simulink model "MIL4L3_SW6_V1_20220211"  (R2018b)
settings: Solver=FixedStepAuto  StartTime=0.0  StopTime=inf  FixedStep=0.001  RelTol=1e-3
PreLoadFcn:
  | A0_MILtest;
undefined symbols (not defined in the file or in its folder): Clb_ICADirect_LaneDisp_StateFive, Clb_ICADirect_LaneDisp_StateFour, Clb_ICADirect_LaneDisp_StateOne, Clb_ICADirect_LaneDisp_StateThree, Clb_ICADirect_LaneDisp_StateTwo, Clb_ICADirect_LaneDisp_StateZero, Clb_ICADirect_LaneDispSW, Clb_ICADirect_TrnLghtsCom_Switch, Clb_ICADirect_TrnLghtsCom_Value, Clb_ICADirect_TrnLghtsCrtl_Inhb, IMAP_Clb_ACU_Driver_Belt, IMAP_Clb_ACU_Driver_Belt_Over, IMAP_Clb_ACU_Passenger_Belt, IMAP_Clb_ACU_Passenger_Belt_Over, IMAP_Clb_ACU_RearLeft_Belt, IMAP_Clb_ACU_RearLeft_Belt_Over, IMAP_Clb_ACU_RearMiddle_Belt, IMAP_Clb_ACU_RearMiddle_Belt_Over, IMAP_Clb_ACU_RearRight_Belt, IMAP_Clb_ACU_RearRight_Belt_Over, IMAP_Clb_AEB_Switch, IMAP_Clb_AEB_Switch_Over, IMAP_Clb_ALC_TLC_Mode, IMAP_Clb_ALC_TLC_Mode_Over, IMAP_Clb_BCM_Battery_Voltage, IMAP_Clb_BCM_Battery_Voltage_Over, IMAP_Clb_BCM_BrakeLamp_State, IMAP_Clb_BCM_BrakeLamp_State_Over, IMAP_Clb_BCM_CHMSL_Status, IMAP_Clb_BCM_CHMSL_Status_Over, IMAP_Clb_BCM_Door_Lock_State, IMAP_Clb_BCM_Door_Lock_State_Over, IMAP_Clb_BCM_FrontWiper_State, IMAP_Clb_BCM_FrontWiper_State_Over, IMAP_Clb_BCM_FrontWiper_Switch, IMAP_Clb_BCM_FrontWiper_Switch_Over, IMAP_Clb_BCM_HazardLamp, IMAP_Clb_BCM_HazardLamp_Over, IMAP_Clb_BCM_HazardLamp_Switch, IMAP_Clb_BCM_HazardLamp_Switch_Over, IMAP_Clb_BCM_HighBeam_State, IMAP_Clb_BCM_HighBeam_State_Over, IMAP_Clb_BCM_Ignition_State, IMAP_Clb_BCM_Ignition_State_Over, IMAP_Clb_BCM_IHBC_Enabled, IMAP_Clb_BCM_IHBC_Enabled_Over, IMAP_Clb_BCM_Left_Light, IMAP_Clb_BCM_Left_Light_Over, IMAP_Clb_BCM_LeftTurn_Switch, IMAP_Clb_BCM_LeftTurn_Switch_Over, IMAP_Clb_BCM_LF_Door_State, IMAP_Clb_BCM_LF_Door_State_Over, IMAP_Clb_BCM_LowBeam_State, IMAP_Clb_BCM_LowBeam_State_Over, IMAP_Clb_BCM_LR_Door_State, IMAP_Clb_BCM_LR_Door_State_Over, IMAP_Clb_BCM_RF_Door_State, IMAP_Clb_BCM_RF_Door_State_Over, IMAP_Clb_BCM_Right_Light, IMAP_Clb_BCM_Right_Light_Over ... (+547)
libraries: CarMaker4SL x2153, simulink x292, dspstat3 x3, canmsglib x2, simulink_extras x1
(part 15 of 52)

== system MIL4L3_SW6_V1_20220211/CarMaker/VehicleControl/SDFADataLog/Subsystem113 ==
  BusCreator : BusCreator  Inputs=10
  Data Type Conversion{1..3,92} (4 alike) : DataTypeConversion  OutDataTypeStr=single
  Ground{,1..5} (6 alike) : Ground
  Read CM Dict1 : CarMaker4SL/Read CM Dict  xname=User.IO.Out.YAcceleration_S1_002  xsync=off
  Read CM Dict2 : CarMaker4SL/Read CM Dict  xname=User.IO.Out.YAcceleration_S1_003  xsync=off
  Read CM Dict3 : CarMaker4SL/Read CM Dict  xname=User.IO.Out.YAcceleration_S1_004  xsync=off
  Read CM Dict5 : CarMaker4SL/Read CM Dict  xname=User.IO.Out.YAcceleration_S1_001  xsync=off
  RBtar_Yacceleration : Outport
  wires:
  Data Type Conversion1/1 -> BusCreator/2
  Data Type Conversion92/1 -> BusCreator/1
  Data Type Conversion3/1 -> BusCreator/4
  Data Type Conversion2/1 -> BusCreator/3
  BusCreator/1 -> RBtar_Yacceleration/1
  Read CM Dict3/1 -> Data Type Conversion3/1
  Read CM Dict2/1 -> Data Type Conversion2/1
  Read CM Dict1/1 -> Data Type Conversion1/1
  Read CM Dict5/1 -> Data Type Conversion92/1
  Ground/1 -> BusCreator/5
  Ground1/1 -> BusCreator/6
  Ground2/1 -> BusCreator/7
  Ground3/1 -> BusCreator/8
  Ground4/1 -> BusCreator/9
  Ground5/1 -> BusCreator/10

== system MIL4L3_SW6_V1_20220211/CarMaker/VehicleControl/SDFADataLog/Subsystem114 ==
  BusCreator : BusCreator  Inputs=10
  Data Type Conversion{1..3,92} (4 alike) : DataTypeConversion  OutDataTypeStr=single
  Ground{,1..5} (6 alike) : Ground
  Read CM Dict1 : CarMaker4SL/Read CM Dict  xname=User.IO.Out.Width_S1_002  xsync=off
  Read CM Dict2 : CarMaker4SL/Read CM Dict  xname=User.IO.Out.Width_S1_003  xsync=off
  Read CM Dict3 : CarMaker4SL/Read CM Dict  xname=User.IO.Out.Width_S1_004  xsync=off
  Read CM Dict5 : CarMaker4SL/Read CM Dict  xname=User.IO.Out.Width_S1_001  xsync=off
  RBtar_Width : Outport
  wires:
  Data Type Conversion2/1 -> BusCreator/3
  Data Type Conversion3/1 -> BusCreator/4
  Data Type Conversion1/1 -> BusCreator/2
  Data Type Conversion92/1 -> BusCreator/1
  Ground5/1 -> BusCreator/10
  Ground4/1 -> BusCreator/9
  Ground3/1 -> BusCreator/8
  Ground2/1 -> BusCreator/7
  Ground1/1 -> BusCreator/6
  Ground/1 -> BusCreator/5
  Read CM Dict5/1 -> Data Type Conversion92/1
  Read CM Dict1/1 -> Data Type Conversion1/1
  Read CM Dict2/1 -> Data Type Conversion2/1
  Read CM Dict3/1 -> Data Type Conversion3/1
  BusCreator/1 -> RBtar_Width/1

== system MIL4L3_SW6_V1_20220211/CarMaker/VehicleControl/SDFADataLog/Subsystem115 ==
  BusCreator : BusCreator  Inputs=10
  Data Type Conversion{1..3,92} (4 alike) : DataTypeConversion  OutDataTypeStr=single
  Ground{,1..5} (6 alike) : Ground
  Read CM Dict1 : CarMaker4SL/Read CM Dict  xname=User.IO.Out.Length_S1_002  xsync=off
  Read CM Dict2 : CarMaker4SL/Read CM Dict  xname=User.IO.Out.Length_S1_003  xsync=off
  Read CM Dict3 : CarMaker4SL/Read CM Dict  xname=User.IO.Out.Length_S1_004  xsync=off
  Read CM Dict5 : CarMaker4SL/Read CM Dict  xname=User.IO.Out.Length_S1_001  xsync=off
  RBtar_Length : Outport
  wires:
  Data Type Conversion2/1 -> BusCreator/3
  Data Type Conversion3/1 -> BusCreator/4
  Data Type Conversion92/1 -> BusCreator/1
  Data Type Conversion1/1 -> BusCreator/2
  BusCreator/1 -> RBtar_Length/1
  Read CM Dict3/1 -> Data Type Conversion3/1
  Read CM Dict2/1 -> Data Type Conversion2/1
  Read CM Dict1/1 -> Data Type Conversion1/1
  Read CM Dict5/1 -> Data Type Conversion92/1
  Ground/1 -> BusCreator/5
  Ground1/1 -> BusCreator/6
  Ground2/1 -> BusCreator/7
  Ground3/1 -> BusCreator/8
  Ground4/1 -> BusCreator/9
  Ground5/1 -> BusCreator/10

== system MIL4L3_SW6_V1_20220211/CarMaker/VehicleControl/SDFADataLog/Subsystem116 ==
  BusCreator : BusCreator  Inputs=10
  Data Type Conversion{1..3,92} (4 alike) : DataTypeConversion  OutDataTypeStr=single
  Ground{,1..5} (6 alike) : Ground
  Read CM Dict1 : CarMaker4SL/Read CM Dict  xname=User.IO.Out.Orientation_S1_002  xsync=off
  Read CM Dict2 : CarMaker4SL/Read CM Dict  xname=User.IO.Out.Orientation_S1_003  xsync=off
  Read CM Dict3 : CarMaker4SL/Read CM Dict  xname=User.IO.Out.Orientation_S1_004  xsync=off
  Read CM Dict5 : CarMaker4SL/Read CM Dict  xname=User.IO.Out.Orientation_S1_001  xsync=off
  RBtar_Orientation : Outport
  wires:
  Data Type Conversion92/1 -> BusCreator/1
  Data Type Conversion3/1 -> BusCreator/4
  Data Type Conversion2/1 -> BusCreator/3
  Data Type Conversion1/1 -> BusCreator/2
  Ground5/1 -> BusCreator/10
  Ground4/1 -> BusCreator/9
  Ground3/1 -> BusCreator/8
  Ground2/1 -> BusCreator/7
  Ground1/1 -> BusCreator/6
  Ground/1 -> BusCreator/5
  Read CM Dict5/1 -> Data Type Conversion92/1
  Read CM Dict1/1 -> Data Type Conversion1/1
  Read CM Dict2/1 -> Data Type Conversion2/1
  Read CM Dict3/1 -> Data Type Conversion3/1
  BusCreator/1 -> RBtar_Orientation/1

== system MIL4L3_SW6_V1_20220211/CarMaker/VehicleControl/SDFADataLog/Subsystem117 ==
  BusCreator : BusCreator  Inputs=10
  Data Type Conversion{1..3,92} (4 alike) : DataTypeConversion  OutDataTypeStr=single
  Ground{,1..5} (6 alike) : Ground
  Read CM Dict1 : CarMaker4SL/Read CM Dict  xname=User.IO.Out.ExistenceProbability_S1_002  xsync=off
  Read CM Dict2 : CarMaker4SL/Read CM Dict  xname=User.IO.Out.ExistenceProbability_S1_003  xsync=off
  Read CM Dict3 : CarMaker4SL/Read CM Dict  xname=User.IO.Out.ExistenceProbability_S1_004  xsync=off
  Read CM Dict5 : CarMaker4SL/Read CM Dict  xname=User.IO.Out.ExistenceProbability_S1_001  xsync=off
  RBtar_ExistenceProbability : Outport
  wires:
  Data Type Conversion3/1 -> BusCreator/4
  Data Type Conversion2/1 -> BusCreator/3
  Data Type Conversion92/1 -> BusCreator/1
  Data Type Conversion1/1 -> BusCreator/2
  BusCreator/1 -> RBtar_ExistenceProbability/1
  Read CM Dict3/1 -> Data Type Conversion3/1
  Read CM Dict2/1 -> Data Type Conversion2/1
  Read CM Dict1/1 -> Data Type Conversion1/1
  Read CM Dict5/1 -> Data Type Conversion92/1
  Ground/1 -> BusCreator/5
  Ground1/1 -> BusCreator/6
  Ground2/1 -> BusCreator/7
  Ground3/1 -> BusCreator/8
  Ground4/1 -> BusCreator/9
  Ground5/1 -> BusCreator/10

== system MIL4L3_SW6_V1_20220211/CarMaker/VehicleControl/SDFADataLog/Subsystem118 ==
  BusCreator : BusCreator  Inputs=10
  Data Type Conversion{1..3,92} (4 alike) : DataTypeConversion  OutDataTypeStr=uint8
  Ground{,1..5} (6 alike) : Ground
  Read CM Dict1 : CarMaker4SL/Read CM Dict  xname=User.IO.Out.ClassHighest_S1_002  xsync=off
  Read CM Dict2 : CarMaker4SL/Read CM Dict  xname=User.IO.Out.ClassHighest_S1_003  xsync=off
  Read CM Dict3 : CarMaker4SL/Read CM Dict  xname=User.IO.Out.ClassHighest_S1_004  xsync=off
  Read CM Dict5 : CarMaker4SL/Read CM Dict  xname=User.IO.Out.ClassHighest_S1_001  xsync=off
  RBtar_Class : Outport
  wires:
  Data Type Conversion1/1 -> BusCreator/2
  Data Type Conversion2/1 -> BusCreator/3
  Data Type Conversion3/1 -> BusCreator/4
  Data Type Conversion92/1 -> BusCreator/1
  Ground5/1 -> BusCreator/10
  Ground4/1 -> BusCreator/9
  Ground3/1 -> BusCreator/8
  Ground2/1 -> BusCreator/7
  Ground1/1 -> BusCreator/6
  Ground/1 -> BusCreator/5
  Read CM Dict5/1 -> Data Type Conversion92/1
  Read CM Dict1/1 -> Data Type Conversion1/1
  Read CM Dict2/1 -> Data Type Conversion2/1
  Read CM Dict3/1 -> Data Type Conversion3/1
  BusCreator/1 -> RBtar_Class/1

== system MIL4L3_SW6_V1_20220211/CarMaker/VehicleControl/SDFADataLog/Subsystem119 ==
  BusCreator : BusCreator  Inputs=10
  Data Type Conversion{1..3,92} (4 alike) : DataTypeConversion  OutDataTypeStr=single
  Ground{,1..5} (6 alike) : Ground
  Read CM Dict1 : CarMaker4SL/Read CM Dict  xname=User.IO.Out.ReferencePoint_S1_002  xsync=off
  Read CM Dict2 : CarMaker4SL/Read CM Dict  xname=User.IO.Out.ReferencePoint_S1_003  xsync=off
  Read CM Dict3 : CarMaker4SL/Read CM Dict  xname=User.IO.Out.ReferencePoint_S1_004  xsync=off
  Read CM Dict5 : CarMaker4SL/Read CM Dict  xname=User.IO.Out.ReferencePoint_S1_001  xsync=off
  RBtar_ReferencePoint : Outport
  wires:
  Data Type Conversion3/1 -> BusCreator/4
  Data Type Conversion2/1 -> BusCreator/3
  Data Type Conversion92/1 -> BusCreator/1
  Data Type Conversion1/1 -> BusCreator/2
  BusCreator/1 -> RBtar_ReferencePoint/1
  Read CM Dict3/1 -> Data Type Conversion3/1
  Read CM Dict2/1 -> Data Type Conversion2/1
  Read CM Dict1/1 -> Data Type Conversion1/1
  Read CM Dict5/1 -> Data Type Conversion92/1
  Ground/1 -> BusCreator/5
  Ground1/1 -> BusCreator/6
  Ground2/1 -> BusCreator/7
  Ground3/1 -> BusCreator/8
  Ground4/1 -> BusCreator/9
  Ground5/1 -> BusCreator/10

== system MIL4L3_SW6_V1_20220211/CarMaker/VehicleControl/SDFADataLog/Subsystem12 ==
  Bus Creator : BusCreator  Inputs=20
  Ground{,1..15} (16 alike) : Ground
  Read CM Dict : CarMaker4SL/Read CM Dict  xname=User.IO.Out.IFC_obj01_Rel_VxStdDevValid  xsync=off
  Read CM Dict1 : CarMaker4SL/Read CM Dict  xname=User.IO.Out.IFC_obj02_Rel_VxStdDevValid  xsync=off
  Read CM Dict2 : CarMaker4SL/Read CM Dict  xname=User.IO.Out.IFC_obj03_Rel_VxStdDevValid  xsync=off
  Read CM Dict3 : CarMaker4SL/Read CM Dict  xname=User.IO.Out.IFC_obj04_Rel_VxStdDevValid  xsync=off
  obj_Rel_VxStdDevValid : Outport
  wires:
  Bus Creator/1 -> obj_Rel_VxStdDevValid/1
  Ground15/1 -> Bus Creator/20
  Ground11/1 -> Bus Creator/16
  Ground14/1 -> Bus Creator/19
  Ground12/1 -> Bus Creator/17
  Ground3/1 -> Bus Creator/8
  Ground1/1 -> Bus Creator/6
  Read CM Dict1/1 -> Bus Creator/2
  Read CM Dict/1 -> Bus Creator/1
  Ground6/1 -> Bus Creator/11
  Ground10/1 -> Bus Creator/15
  Ground13/1 -> Bus Creator/18
  Ground2/1 -> Bus Creator/7
  Ground/1 -> Bus Creator/5
  Ground7/1 -> Bus Creator/12
  Read CM Dict3/1 -> Bus Creator/4
  Ground4/1 -> Bus Creator/9
  Ground9/1 -> Bus Creator/14
  Ground5/1 -> Bus Creator/10
  Ground8/1 -> Bus Creator/13
  Read CM Dict2/1 -> Bus Creator/3

== system MIL4L3_SW6_V1_20220211/CarMaker/VehicleControl/SDFADataLog/Subsystem120 ==
  BusCreator : BusCreator  Inputs=10
  Data Type Conversion{1..3,92} (4 alike) : DataTypeConversion  OutDataTypeStr=single
  Ground{,1..5} (6 alike) : Ground
  Read CM Dict1 : CarMaker4SL/Read CM Dict  xname=User.IO.Out.MovingState_S1_002  xsync=off
  Read CM Dict2 : CarMaker4SL/Read CM Dict  xname=User.IO.Out.MovingState_S1_003  xsync=off
  Read CM Dict3 : CarMaker4SL/Read CM Dict  xname=User.IO.Out.MovingState_S1_004  xsync=off
  Read CM Dict5 : CarMaker4SL/Read CM Dict  xname=User.IO.Out.MovingState_S1_001  xsync=off
  RBtar_MovingState : Outport
  wires:
  Data Type Conversion2/1 -> BusCreator/3
  Data Type Conversion92/1 -> BusCreator/1
  Data Type Conversion3/1 -> BusCreator/4
  Data Type Conversion1/1 -> BusCreator/2
  Ground5/1 -> BusCreator/10
  Ground4/1 -> BusCreator/9
  Ground3/1 -> BusCreator/8
  Ground2/1 -> BusCreator/7
  Ground1/1 -> BusCreator/6
  Ground/1 -> BusCreator/5
  Read CM Dict5/1 -> Data Type Conversion92/1
  Read CM Dict1/1 -> Data Type Conversion1/1
  Read CM Dict2/1 -> Data Type Conversion2/1
  Read CM Dict3/1 -> Data Type Conversion3/1
  BusCreator/1 -> RBtar_MovingState/1

== system MIL4L3_SW6_V1_20220211/CarMaker/VehicleControl/SDFADataLog/Subsystem13 ==
  BusCreator : BusCreator  Inputs=24
  Constant{,1..3} (4 alike) : Constant  Value=0
  Ground{,1..19} (20 alike) : Ground
  Read CM Dict : CarMaker4SL/Read CM Dict  Commented=on  xname=User.IO.Out.BrakingAllowed_00  xsync=off
  Read CM Dict1 : CarMaker4SL/Read CM Dict  Commented=on  xname=User.IO.Out.BrakingAllowed_01  xsync=off
  Read CM Dict2 : CarMaker4SL/Read CM Dict  Commented=on  xname=User.IO.Out.BrakingAllowed_02  xsync=off
  Read CM Dict3 : CarMaker4SL/Read CM Dict  Commented=on  xname=User.IO.Out.BrakingAllowed_03  xsync=off
  BrakingAllowed : Outport
  wires:
  Constant3/1 -> BusCreator/4
  Ground19/1 -> BusCreator/24
  Ground18/1 -> BusCreator/23
  Ground5/1 -> BusCreator/10
  Ground3/1 -> BusCreator/8
  Ground9/1 -> BusCreator/14
  BusCreator/1 -> BrakingAllowed/1
  Ground11/1 -> BusCreator/16
  Ground8/1 -> BusCreator/13
  Ground7/1 -> BusCreator/12
  Ground15/1 -> BusCreator/18
  Ground1/1 -> BusCreator/6
  Ground/1 -> BusCreator/5
  Ground13/1 -> BusCreator/22
  Ground4/1 -> BusCreator/9
  Ground17/1 -> BusCreator/20
  Constant/1 -> BusCreator/1
  Ground10/1 -> BusCreator/15
  Constant2/1 -> BusCreator/3
  Ground6/1 -> BusCreator/11
  Constant1/1 -> BusCreator/2
  Ground2/1 -> BusCreator/7
  Ground14/1 -> BusCreator/17
  Ground16/1 -> BusCreator/19
  Ground12/1 -> BusCreator/21

== system MIL4L3_SW6_V1_20220211/CarMaker/VehicleControl/SDFADataLog/Subsystem14 ==
  BusCreator : BusCreator  Inputs=24
  Ground{,1..19} (20 alike) : Ground
  Read CM Dict : CarMaker4SL/Read CM Dict  xname=User.IO.Out.RadarCrossSection_00  xsync=off
  Read CM Dict1 : CarMaker4SL/Read CM Dict  xname=User.IO.Out.RadarCrossSection_01  xsync=off
  Read CM Dict2 : CarMaker4SL/Read CM Dict  xname=User.IO.Out.RadarCrossSection_02  xsync=off
  Read CM Dict3 : CarMaker4SL/Read CM Dict  xname=User.IO.Out.RadarCrossSection_03  xsync=off
  RadarCrossSection : Outport
  wires:
  Ground12/1 -> BusCreator/21
  Ground16/1 -> BusCreator/19
  Ground14/1 -> BusCreator/17
  Ground2/1 -> BusCreator/7
  Read CM Dict1/1 -> BusCreator/2
  Ground6/1 -> BusCreator/11
  Read CM Dict2/1 -> BusCreator/3
  Ground10/1 -> BusCreator/15
  Read CM Dict/1 -> BusCreator/1
  Ground17/1 -> BusCreator/20
  Ground4/1 -> BusCreator/9
  Ground13/1 -> BusCreator/22
  Ground/1 -> BusCreator/5
  Ground1/1 -> BusCreator/6
  Ground15/1 -> BusCreator/18
  Ground7/1 -> BusCreator/12
  Ground8/1 -> BusCreator/13
  Ground11/1 -> BusCreator/16
  BusCreator/1 -> RadarCrossSection/1
  Ground9/1 -> BusCreator/14
  Ground3/1 -> BusCreator/8
  Ground5/1 -> BusCreator/10
  Ground18/1 -> BusCreator/23
  Ground19/1 -> BusCreator/24
  Read CM Dict3/1 -> BusCreator/4

== system MIL4L3_SW6_V1_20220211/CarMaker/VehicleControl/SDFADataLog/Subsystem149 ==
  Bus Creator : BusCreator  Inputs=20
  Ground{,1..15} (16 alike) : Ground
  Read CM Dict : CarMaker4SL/Read CM Dict  xname=User.IO.Out.IFC_obj01_ExistProb  xsync=off
  Read CM Dict1 : CarMaker4SL/Read CM Dict  xname=User.IO.Out.IFC_obj02_ExistProb  xsync=off
  Read CM Dict2 : CarMaker4SL/Read CM Dict  xname=User.IO.Out.IFC_obj03_ExistProb  xsync=off
  Read CM Dict3 : CarMaker4SL/Read CM Dict  xname=User.IO.Out.IFC_obj04_ExistProb  xsync=off
  obj_ExistProb : Outport
  wires:
  Bus Creator/1 -> obj_ExistProb/1
  Ground15/1 -> Bus Creator/20
  Ground11/1 -> Bus Creator/16
  Ground14/1 -> Bus Creator/19
  Ground12/1 -> Bus Creator/17
  Ground3/1 -> Bus Creator/8
  Ground1/1 -> Bus Creator/6
  Read CM Dict1/1 -> Bus Creator/2
  Read CM Dict/1 -> Bus Creator/1
  Ground6/1 -> Bus Creator/11
  Ground10/1 -> Bus Creator/15
  Ground13/1 -> Bus Creator/18
  Ground2/1 -> Bus Creator/7
  Ground/1 -> Bus Creator/5
  Ground7/1 -> Bus Creator/12
  Read CM Dict3/1 -> Bus Creator/4
  Ground4/1 -> Bus Creator/9
  Ground9/1 -> Bus Creator/14
  Ground5/1 -> Bus Creator/10
  Ground8/1 -> Bus Creator/13
  Read CM Dict2/1 -> Bus Creator/3

== system MIL4L3_SW6_V1_20220211/CarMaker/VehicleControl/SDFADataLog/Subsystem150 ==
  BusCreator : BusCreator  Inputs=24
  Ground{,1..19} (20 alike) : Ground
  Read CM Dict : CarMaker4SL/Read CM Dict  xname=User.IO.Out.AbsoluteLongAcc_00  xsync=off
  Read CM Dict1 : CarMaker4SL/Read CM Dict  xname=User.IO.Out.AbsoluteLongAcc_01  xsync=off
  Read CM Dict2 : CarMaker4SL/Read CM Dict  xname=User.IO.Out.AbsoluteLongAcc_02  xsync=off
  Read CM Dict3 : CarMaker4SL/Read CM Dict  xname=User.IO.Out.AbsoluteLongAcc_03  xsync=off
  AbsoluteLongAcc : Outport
  wires:
  Ground12/1 -> BusCreator/21
  Ground16/1 -> BusCreator/19
  Ground14/1 -> BusCreator/17
  Ground2/1 -> BusCreator/7
  Read CM Dict1/1 -> BusCreator/2
  Ground6/1 -> BusCreator/11
  Read CM Dict2/1 -> BusCreator/3
  Ground10/1 -> BusCreator/15
  Read CM Dict/1 -> BusCreator/1
  Ground17/1 -> BusCreator/20
  Ground4/1 -> BusCreator/9
  Ground13/1 -> BusCreator/22
  Ground/1 -> BusCreator/5
  Ground1/1 -> BusCreator/6
  Ground15/1 -> BusCreator/18
  Ground7/1 -> BusCreator/12
  Ground8/1 -> BusCreator/13
  Ground11/1 -> BusCreator/16
  BusCreator/1 -> AbsoluteLongAcc/1
  Ground9/1 -> BusCreator/14
  Ground3/1 -> BusCreator/8
  Ground5/1 -> BusCreator/10
  Ground18/1 -> BusCreator/23
  Ground19/1 -> BusCreator/24
  Read CM Dict3/1 -> BusCreator/4

== system MIL4L3_SW6_V1_20220211/CarMaker/VehicleControl/SDFADataLog/Subsystem160 ==
  Bus Creator : BusCreator  Inputs=20
  Ground{,1..15} (16 alike) : Ground
  Read CM Dict : CarMaker4SL/Read CM Dict  xname=User.IO.Out.IFC_obj01_Rel_Vx  xsync=off
  Read CM Dict1 : CarMaker4SL/Read CM Dict  xname=User.IO.Out.IFC_obj02_Rel_Vx  xsync=off
  Read CM Dict2 : CarMaker4SL/Read CM Dict  xname=User.IO.Out.IFC_obj03_Rel_Vx  xsync=off
  Read CM Dict3 : CarMaker4SL/Read CM Dict  xname=User.IO.Out.IFC_obj04_Rel_Vx  xsync=off
  obj_Rel_Vx : Outport
  wires:
  Bus Creator/1 -> obj_Rel_Vx/1
  Ground15/1 -> Bus Creator/20
  Ground11/1 -> Bus Creator/16
  Ground14/1 -> Bus Creator/19
  Ground12/1 -> Bus Creator/17
  Ground3/1 -> Bus Creator/8
  Ground1/1 -> Bus Creator/6
  Read CM Dict1/1 -> Bus Creator/2
  Read CM Dict/1 -> Bus Creator/1
  Ground6/1 -> Bus Creator/11
  Ground10/1 -> Bus Creator/15
  Ground13/1 -> Bus Creator/18
  Ground2/1 -> Bus Creator/7
  Ground/1 -> Bus Creator/5
  Ground7/1 -> Bus Creator/12
  Read CM Dict3/1 -> Bus Creator/4
  Ground4/1 -> Bus Creator/9
  Ground9/1 -> Bus Creator/14
  Ground5/1 -> Bus Creator/10
  Ground8/1 -> Bus Creator/13
  Read CM Dict2/1 -> Bus Creator/3

== system MIL4L3_SW6_V1_20220211/CarMaker/VehicleControl/SDFADataLog/Subsystem171 ==
  Bus Creator : BusCreator  Inputs=20
  Ground{,1..15} (16 alike) : Ground
  Read CM Dict : CarMaker4SL/Read CM Dict  xname=User.IO.Out.IFC_obj01_Rel_VxValid  xsync=off
  Read CM Dict1 : CarMaker4SL/Read CM Dict  xname=User.IO.Out.IFC_obj02_Rel_VxValid  xsync=off
  Read CM Dict2 : CarMaker4SL/Read CM Dict  xname=User.IO.Out.IFC_obj03_Rel_VxValid  xsync=off
  Read CM Dict3 : CarMaker4SL/Read CM Dict  xname=User.IO.Out.IFC_obj04_Rel_VxValid  xsync=off
  obj_Rel_VxValid : Outport
  wires:
  Bus Creator/1 -> obj_Rel_VxValid/1
  Ground15/1 -> Bus Creator/20
  Ground11/1 -> Bus Creator/16
  Ground14/1 -> Bus Creator/19
  Ground12/1 -> Bus Creator/17
  Ground3/1 -> Bus Creator/8
  Ground1/1 -> Bus Creator/6
  Read CM Dict1/1 -> Bus Creator/2
  Read CM Dict/1 -> Bus Creator/1
  Ground6/1 -> Bus Creator/11
  Ground10/1 -> Bus Creator/15
  Ground13/1 -> Bus Creator/18
  Ground2/1 -> Bus Creator/7
  Ground/1 -> Bus Creator/5
  Ground7/1 -> Bus Creator/12
  Read CM Dict3/1 -> Bus Creator/4
  Ground4/1 -> Bus Creator/9
  Ground9/1 -> Bus Creator/14
  Ground5/1 -> Bus Creator/10
  Ground8/1 -> Bus Creator/13
  Read CM Dict2/1 -> Bus Creator/3

== system MIL4L3_SW6_V1_20220211/CarMaker/VehicleControl/SDFADataLog/Subsystem174 ==
  BusCreator : BusCreator  Inputs=24
  Constant{1..4} (4 alike) : Constant  Value=0.01
  Define CM Dict_User.IO.Out.LateralDistanceSTD_00 : CarMaker4SL/Define CM Dict  Commented=on  xname=User.IO.Out.LateralDistanceSTD_00  xunit=m  xmono=off  xtype=Double4  xdvaplace=IO_Out  xnstates=0  xfirststate=0  xinitial=0
  Ground{,1..19} (20 alike) : Ground
  LateralDistanceSTD : Outport
  wires:
  Ground18/1 -> BusCreator/23
  Ground19/1 -> BusCreator/24
  BusCreator/1 -> LateralDistanceSTD/1
  Ground8/1 -> BusCreator/13
  Ground5/1 -> BusCreator/10
  Ground3/1 -> BusCreator/8
  Ground/1 -> BusCreator/5
  Ground6/1 -> BusCreator/11
  Ground7/1 -> BusCreator/12
  Ground1/1 -> BusCreator/6
  Ground9/1 -> BusCreator/14
  Ground10/1 -> BusCreator/15
  Ground11/1 -> BusCreator/16
  Ground15/1 -> BusCreator/18
  Ground4/1 -> BusCreator/9
  Ground13/1 -> BusCreator/22
  Ground12/1 -> BusCreator/21
  Ground14/1 -> BusCreator/17
  Ground17/1 -> BusCreator/20
  Ground2/1 -> BusCreator/7
  Ground16/1 -> BusCreator/19
  Constant1/1 -> BusCreator/1
  Constant2/1 -> BusCreator/2
  Constant3/1 -> BusCreator/3
  Constant4/1 -> BusCreator/4

== system MIL4L3_SW6_V1_20220211/CarMaker/VehicleControl/SDFADataLog/Subsystem175 ==
  BusCreator : BusCreator  Inputs=24
  Constant{1..4} (4 alike) : Constant  Value=0.01
  Define CM Dict_User.IO.Out.LongDistanceSTD_00 : CarMaker4SL/Define CM Dict  Commented=on  xname=User.IO.Out.LongDistanceSTD_00  xunit=m  xmono=off  xtype=Double4  xdvaplace=IO_Out  xnstates=0  xfirststate=0  xinitial=0
  Ground{,1..19} (20 alike) : Ground
  Read CM Dict : CarMaker4SL/Read CM Dict  Commented=on  xname=User.IO.Out.LongDistance_00  xsync=off
  LongDistanceSTD : Outport
  wires:
  Constant4/1 -> BusCreator/4
  Constant3/1 -> BusCreator/3
  Constant2/1 -> BusCreator/2
  Constant1/1 -> BusCreator/1
  Ground16/1 -> BusCreator/19
  Ground2/1 -> BusCreator/7
  Ground17/1 -> BusCreator/20
  Ground14/1 -> BusCreator/17
  Ground12/1 -> BusCreator/21
  Ground13/1 -> BusCreator/22
  Ground4/1 -> BusCreator/9
  Ground15/1 -> BusCreator/18
  Ground11/1 -> BusCreator/16
  Ground10/1 -> BusCreator/15
  Ground9/1 -> BusCreator/14
  Ground1/1 -> BusCreator/6
  Ground7/1 -> BusCreator/12
  Ground6/1 -> BusCreator/11
  Ground/1 -> BusCreator/5
  Ground3/1 -> BusCreator/8
  Ground5/1 -> BusCreator/10
  Ground8/1 -> BusCreator/13
  BusCreator/1 -> LongDistanceSTD/1
  Ground19/1 -> BusCreator/24
  Ground18/1 -> BusCreator/23

== system MIL4L3_SW6_V1_20220211/CarMaker/VehicleControl/SDFADataLog/Subsystem176 ==
  BusCreator : BusCreator  Inputs=24
  Constant{,1..3} (4 alike) : Constant  Value=0.01
  Ground{,1..19} (20 alike) : Ground
  AbsoluteLongAccSTD : Outport
  wires:
  Constant3/1 -> BusCreator/4
  Ground19/1 -> BusCreator/24
  Ground18/1 -> BusCreator/23
  Ground5/1 -> BusCreator/10
  Ground3/1 -> BusCreator/8
  Ground9/1 -> BusCreator/14
  BusCreator/1 -> AbsoluteLongAccSTD/1
  Ground11/1 -> BusCreator/16
  Ground8/1 -> BusCreator/13
  Ground7/1 -> BusCreator/12
  Ground15/1 -> BusCreator/18
  Ground1/1 -> BusCreator/6
  Ground/1 -> BusCreator/5
  Ground13/1 -> BusCreator/22
  Ground4/1 -> BusCreator/9
  Ground17/1 -> BusCreator/20
  Constant/1 -> BusCreator/1
  Ground10/1 -> BusCreator/15
  Constant2/1 -> BusCreator/3
  Ground6/1 -> BusCreator/11
  Constant1/1 -> BusCreator/2
  Ground2/1 -> BusCreator/7
  Ground14/1 -> BusCreator/17
  Ground16/1 -> BusCreator/19
  Ground12/1 -> BusCreator/21

== system MIL4L3_SW6_V1_20220211/CarMaker/VehicleControl/SDFADataLog/Subsystem177 ==
  BusCreator : BusCreator  Inputs=24
  Constant{,1..3} (4 alike) : Constant  Value=0.01
  Ground{,1..19} (20 alike) : Ground
  AbsoluteLatVeloSTD : Outport
  wires:
  Constant3/1 -> BusCreator/4
  Ground19/1 -> BusCreator/24
  Ground18/1 -> BusCreator/23
  Ground5/1 -> BusCreator/10
  Ground3/1 -> BusCreator/8
  Ground9/1 -> BusCreator/14
  BusCreator/1 -> AbsoluteLatVeloSTD/1
  Ground11/1 -> BusCreator/16
  Ground8/1 -> BusCreator/13
  Ground7/1 -> BusCreator/12
  Ground15/1 -> BusCreator/18
  Ground1/1 -> BusCreator/6
  Ground/1 -> BusCreator/5
  Ground13/1 -> BusCreator/22
  Ground4/1 -> BusCreator/9
  Ground17/1 -> BusCreator/20
  Constant/1 -> BusCreator/1
  Ground10/1 -> BusCreator/15
  Constant2/1 -> BusCreator/3
  Ground6/1 -> BusCreator/11
  Constant1/1 -> BusCreator/2
  Ground2/1 -> BusCreator/7
  Ground14/1 -> BusCreator/17
  Ground16/1 -> BusCreator/19
  Ground12/1 -> BusCreator/21

== system MIL4L3_SW6_V1_20220211/CarMaker/VehicleControl/SDFADataLog/Subsystem178 ==
  BusCreator : BusCreator  Inputs=24
  Constant{,1..3} (4 alike) : Constant  Value=0.01
  Ground{,1..19} (20 alike) : Ground
  AbsLatAccSTD : Outport
  wires:
  Constant3/1 -> BusCreator/4
  Ground19/1 -> BusCreator/24
  Ground18/1 -> BusCreator/23
  Ground5/1 -> BusCreator/10
  Ground3/1 -> BusCreator/8
  Ground9/1 -> BusCreator/14
  BusCreator/1 -> AbsLatAccSTD/1
  Ground11/1 -> BusCreator/16
  Ground8/1 -> BusCreator/13
  Ground7/1 -> BusCreator/12
  Ground15/1 -> BusCreator/18
  Ground1/1 -> BusCreator/6
  Ground/1 -> BusCreator/5
  Ground13/1 -> BusCreator/22
  Ground4/1 -> BusCreator/9
  Ground17/1 -> BusCreator/20
  Constant/1 -> BusCreator/1
  Ground10/1 -> BusCreator/15
  Constant2/1 -> BusCreator/3
  Ground6/1 -> BusCreator/11
  Constant1/1 -> BusCreator/2
  Ground2/1 -> BusCreator/7
  Ground14/1 -> BusCreator/17
  Ground16/1 -> BusCreator/19
  Ground12/1 -> BusCreator/21

== system MIL4L3_SW6_V1_20220211/CarMaker/VehicleControl/SDFADataLog/Subsystem179 ==
  BusCreator : BusCreator  Inputs=24
  Constant{,1..3} (4 alike) : Constant  Value=0.01
  Ground{,1..19} (20 alike) : Ground
  LengthSTD : Outport
  wires:
  Constant3/1 -> BusCreator/4
  Ground19/1 -> BusCreator/24
  Ground18/1 -> BusCreator/23
  Ground5/1 -> BusCreator/10
  Ground3/1 -> BusCreator/8
  Ground9/1 -> BusCreator/14
  BusCreator/1 -> LengthSTD/1
  Ground11/1 -> BusCreator/16
  Ground8/1 -> BusCreator/13
  Ground7/1 -> BusCreator/12
  Ground15/1 -> BusCreator/18
  Ground1/1 -> BusCreator/6
  Ground/1 -> BusCreator/5
  Ground13/1 -> BusCreator/22
  Ground4/1 -> BusCreator/9
  Ground17/1 -> BusCreator/20
  Constant/1 -> BusCreator/1
  Ground10/1 -> BusCreator/15
  Constant2/1 -> BusCreator/3
  Ground6/1 -> BusCreator/11
  Constant1/1 -> BusCreator/2
  Ground2/1 -> BusCreator/7
  Ground14/1 -> BusCreator/17
  Ground16/1 -> BusCreator/19
  Ground12/1 -> BusCreator/21

== system MIL4L3_SW6_V1_20220211/CarMaker/VehicleControl/SDFADataLog/Subsystem180 ==
  BusCreator : BusCreator  Inputs=24
  Constant{,1..3} (4 alike) : Constant  Value=0.01
  Ground{,1..19} (20 alike) : Ground
  WidhSTD : Outport
  wires:
  Constant3/1 -> BusCreator/4
  Ground19/1 -> BusCreator/24
  Ground18/1 -> BusCreator/23
  Ground5/1 -> BusCreator/10
  Ground3/1 -> BusCreator/8
  Ground9/1 -> BusCreator/14
  BusCreator/1 -> WidhSTD/1
  Ground11/1 -> BusCreator/16
  Ground8/1 -> BusCreator/13
  Ground7/1 -> BusCreator/12
  Ground15/1 -> BusCreator/18
  Ground1/1 -> BusCreator/6
  Ground/1 -> BusCreator/5
  Ground13/1 -> BusCreator/22
  Ground4/1 -> BusCreator/9
  Ground17/1 -> BusCreator/20
  Constant/1 -> BusCreator/1
  Ground10/1 -> BusCreator/15
  Constant2/1 -> BusCreator/3
  Ground6/1 -> BusCreator/11
  Constant1/1 -> BusCreator/2
  Ground2/1 -> BusCreator/7
  Ground14/1 -> BusCreator/17
  Ground16/1 -> BusCreator/19
  Ground12/1 -> BusCreator/21

== system MIL4L3_SW6_V1_20220211/CarMaker/VehicleControl/SDFADataLog/Subsystem181 ==
  BusCreator : BusCreator  Inputs=24
  Constant{,1..3} (4 alike) : Constant  Value=0.01
  Ground{,1..19} (20 alike) : Ground
  HeightSTD : Outport
  wires:
  Constant3/1 -> BusCreator/4
  Ground19/1 -> BusCreator/24
  Ground18/1 -> BusCreator/23
  Ground5/1 -> BusCreator/10
  Ground3/1 -> BusCreator/8
  Ground9/1 -> BusCreator/14
  BusCreator/1 -> HeightSTD/1
  Ground11/1 -> BusCreator/16
  Ground8/1 -> BusCreator/13
  Ground7/1 -> BusCreator/12
  Ground15/1 -> BusCreator/18
  Ground1/1 -> BusCreator/6
  Ground/1 -> BusCreator/5
  Ground13/1 -> BusCreator/22
  Ground4/1 -> BusCreator/9
  Ground17/1 -> BusCreator/20
  Constant/1 -> BusCreator/1
  Ground10/1 -> BusCreator/15
  Constant2/1 -> BusCreator/3
  Ground6/1 -> BusCreator/11
  Constant1/1 -> BusCreator/2
  Ground2/1 -> BusCreator/7
  Ground14/1 -> BusCreator/17
  Ground16/1 -> BusCreator/19
  Ground12/1 -> BusCreator/21

== system MIL4L3_SW6_V1_20220211/CarMaker/VehicleControl/SDFADataLog/Subsystem182 ==
  BusCreator : BusCreator  Inputs=24
  Ground{,1..19} (20 alike) : Ground
  Read CM Dict : CarMaker4SL/Read CM Dict  xname=User.IO.Out.AbsoluteLatVelo_00  xsync=off
  Read CM Dict1 : CarMaker4SL/Read CM Dict  xname=User.IO.Out.AbsoluteLatVelo_01  xsync=off
  Read CM Dict2 : CarMaker4SL/Read CM Dict  xname=User.IO.Out.AbsoluteLatVelo_02  xsync=off
  Read CM Dict3 : CarMaker4SL/Read CM Dict  xname=User.IO.Out.AbsoluteLatVelo_03  xsync=off
  AbsoluteLatVelo : Outport
  wires:
  Ground12/1 -> BusCreator/21
  Ground16/1 -> BusCreator/19
  Ground14/1 -> BusCreator/17
  Ground2/1 -> BusCreator/7
  Read CM Dict1/1 -> BusCreator/2
  Ground6/1 -> BusCreator/11
  Read CM Dict2/1 -> BusCreator/3
  Ground10/1 -> BusCreator/15
  Read CM Dict/1 -> BusCreator/1
  Ground17/1 -> BusCreator/20
  Ground4/1 -> BusCreator/9
  Ground13/1 -> BusCreator/22
  Ground/1 -> BusCreator/5
  Ground1/1 -> BusCreator/6
  Ground15/1 -> BusCreator/18
  Ground7/1 -> BusCreator/12
  Ground8/1 -> BusCreator/13
  Ground11/1 -> BusCreator/16
  BusCreator/1 -> AbsoluteLatVelo/1
  Ground9/1 -> BusCreator/14
  Ground3/1 -> BusCreator/8
  Ground5/1 -> BusCreator/10
  Ground18/1 -> BusCreator/23
  Ground19/1 -> BusCreator/24
  Read CM Dict3/1 -> BusCreator/4

== system MIL4L3_SW6_V1_20220211/CarMaker/VehicleControl/SDFADataLog/Subsystem183 ==
  BusCreator : BusCreator  Inputs=24
  Constant{,1..3} (4 alike) : Constant  Value=0.01
  Ground{,1..19} (20 alike) : Ground
  YawSTD : Outport
  wires:
  Constant3/1 -> BusCreator/4
  Ground19/1 -> BusCreator/24
  Ground18/1 -> BusCreator/23
  Ground5/1 -> BusCreator/10
  Ground3/1 -> BusCreator/8
  Ground9/1 -> BusCreator/14
  BusCreator/1 -> YawSTD/1
  Ground11/1 -> BusCreator/16
  Ground8/1 -> BusCreator/13
  Ground7/1 -> BusCreator/12
  Ground15/1 -> BusCreator/18
  Ground1/1 -> BusCreator/6
  Ground/1 -> BusCreator/5
  Ground13/1 -> BusCreator/22
  Ground4/1 -> BusCreator/9
  Ground17/1 -> BusCreator/20
  Constant/1 -> BusCreator/1
  Ground10/1 -> BusCreator/15
  Constant2/1 -> BusCreator/3
  Ground6/1 -> BusCreator/11
  Constant1/1 -> BusCreator/2
  Ground2/1 -> BusCreator/7
  Ground14/1 -> BusCreator/17
  Ground16/1 -> BusCreator/19
  Ground12/1 -> BusCreator/21

== system MIL4L3_SW6_V1_20220211/CarMaker/VehicleControl/SDFADataLog/Subsystem184 ==
  Bus Creator : BusCreator  Inputs=20
  Constant{,1..3} (4 alike) : Constant  Value=0.01
  Ground{,1..15} (16 alike) : Ground
  obj_PhiRightSTD : Outport
  wires:
  Constant2/1 -> Bus Creator/3
  Ground8/1 -> Bus Creator/13
  Ground5/1 -> Bus Creator/10
  Ground9/1 -> Bus Creator/14
  Ground4/1 -> Bus Creator/9
  Constant3/1 -> Bus Creator/4
  Ground7/1 -> Bus Creator/12
  Ground/1 -> Bus Creator/5
  Ground2/1 -> Bus Creator/7
  Ground13/1 -> Bus Creator/18
  Ground10/1 -> Bus Creator/15
  Ground6/1 -> Bus Creator/11
  Constant/1 -> Bus Creator/1
  Constant1/1 -> Bus Creator/2
  Ground1/1 -> Bus Creator/6
  Ground3/1 -> Bus Creator/8
  Ground12/1 -> Bus Creator/17
  Ground14/1 -> Bus Creator/19
  Ground11/1 -> Bus Creator/16
  Ground15/1 -> Bus Creator/20
  Bus Creator/1 -> obj_PhiRightSTD/1

== system MIL4L3_SW6_V1_20220211/CarMaker/VehicleControl/SDFADataLog/Subsystem185 ==
  Bus Creator : BusCreator  Inputs=20
  Constant{,1..3} (4 alike) : Constant  Value=0.01
  Ground{,1..15} (16 alike) : Ground
  obj_WidthSTD : Outport
  wires:
  Constant2/1 -> Bus Creator/3
  Ground8/1 -> Bus Creator/13
  Ground5/1 -> Bus Creator/10
  Ground9/1 -> Bus Creator/14
  Ground4/1 -> Bus Creator/9
  Constant3/1 -> Bus Creator/4
  Ground7/1 -> Bus Creator/12
  Ground/1 -> Bus Creator/5
  Ground2/1 -> Bus Creator/7
  Ground13/1 -> Bus Creator/18
  Ground10/1 -> Bus Creator/15
  Ground6/1 -> Bus Creator/11
  Constant/1 -> Bus Creator/1
  Constant1/1 -> Bus Creator/2
  Ground1/1 -> Bus Creator/6
  Ground3/1 -> Bus Creator/8
  Ground12/1 -> Bus Creator/17
  Ground14/1 -> Bus Creator/19
  Ground11/1 -> Bus Creator/16
  Ground15/1 -> Bus Creator/20
  Bus Creator/1 -> obj_WidthSTD/1

== system MIL4L3_SW6_V1_20220211/CarMaker/VehicleControl/SDFADataLog/Subsystem186 ==
  Bus Creator : BusCreator  Inputs=20
  Constant{,1..3} (4 alike) : Constant  Value=0.01
  Ground{,1..15} (16 alike) : Ground
  obj_abgle_rate_STD : Outport
  wires:
  Constant2/1 -> Bus Creator/3
  Ground8/1 -> Bus Creator/13
  Ground5/1 -> Bus Creator/10
  Ground9/1 -> Bus Creator/14
  Ground4/1 -> Bus Creator/9
  Constant3/1 -> Bus Creator/4
  Ground7/1 -> Bus Creator/12
  Ground/1 -> Bus Creator/5
  Ground2/1 -> Bus Creator/7
  Ground13/1 -> Bus Creator/18
  Ground10/1 -> Bus Creator/15
  Ground6/1 -> Bus Creator/11
  Constant/1 -> Bus Creator/1
  Constant1/1 -> Bus Creator/2
  Ground1/1 -> Bus Creator/6
  Ground3/1 -> Bus Creator/8
  Ground12/1 -> Bus Creator/17
  Ground14/1 -> Bus Creator/19
  Ground11/1 -> Bus Creator/16
  Ground15/1 -> Bus Creator/20
  Bus Creator/1 -> obj_abgle_rate_STD/1

== system MIL4L3_SW6_V1_20220211/CarMaker/VehicleControl/SDFADataLog/Subsystem187 ==
  Bus Creator : BusCreator  Inputs=20
  Constant{,1..3} (4 alike) : Constant  Value=0.01
  Ground{,1..15} (16 alike) : Ground
  obj_HeightSTD : Outport
  wires:
  Constant2/1 -> Bus Creator/3
  Ground8/1 -> Bus Creator/13
  Ground5/1 -> Bus Creator/10
  Ground9/1 -> Bus Creator/14
  Ground4/1 -> Bus Creator/9
  Constant3/1 -> Bus Creator/4
  Ground7/1 -> Bus Creator/12
  Ground/1 -> Bus Creator/5
  Ground2/1 -> Bus Creator/7
  Ground13/1 -> Bus Creator/18
  Ground10/1 -> Bus Creator/15
  Ground6/1 -> Bus Creator/11
  Constant/1 -> Bus Creator/1
  Constant1/1 -> Bus Creator/2
  Ground1/1 -> Bus Creator/6
  Ground3/1 -> Bus Creator/8
  Ground12/1 -> Bus Creator/17
  Ground14/1 -> Bus Creator/19
  Ground11/1 -> Bus Creator/16
  Ground15/1 -> Bus Creator/20
  Bus Creator/1 -> obj_HeightSTD/1

== system MIL4L3_SW6_V1_20220211/CarMaker/VehicleControl/SDFADataLog/Subsystem188 ==
  Bus Creator : BusCreator  Inputs=20
  Constant{,1..3} (4 alike) : Constant  Value=0.01
  Ground{,1..15} (16 alike) : Ground
  obj_LengthSTD : Outport
  wires:
  Constant2/1 -> Bus Creator/3
  Ground8/1 -> Bus Creator/13
  Ground5/1 -> Bus Creator/10
  Ground9/1 -> Bus Creator/14
  Ground4/1 -> Bus Creator/9
  Constant3/1 -> Bus Creator/4
  Ground7/1 -> Bus Creator/12
  Ground/1 -> Bus Creator/5
  Ground2/1 -> Bus Creator/7
  Ground13/1 -> Bus Creator/18
  Ground10/1 -> Bus Creator/15
  Ground6/1 -> Bus Creator/11
  Constant/1 -> Bus Creator/1
  Constant1/1 -> Bus Creator/2
  Ground1/1 -> Bus Creator/6
  Ground3/1 -> Bus Creator/8
  Ground12/1 -> Bus Creator/17
  Ground14/1 -> Bus Creator/19
  Ground11/1 -> Bus Creator/16
  Ground15/1 -> Bus Creator/20
  Bus Creator/1 -> obj_LengthSTD/1

== system MIL4L3_SW6_V1_20220211/CarMaker/VehicleControl/SDFADataLog/Subsystem189 ==
  Bus Creator : BusCreator  Inputs=20
  Constant{,1..3} (4 alike) : Constant  Value=0.01
  Ground{,1..15} (16 alike) : Ground
  obj_HeadingSTD : Outport
  wires:
  Constant2/1 -> Bus Creator/3
  Ground8/1 -> Bus Creator/13
  Ground5/1 -> Bus Creator/10
  Ground9/1 -> Bus Creator/14
  Ground4/1 -> Bus Creator/9
  Constant3/1 -> Bus Creator/4
  Ground7/1 -> Bus Creator/12
  Ground/1 -> Bus Creator/5
  Ground2/1 -> Bus Creator/7
  Ground13/1 -> Bus Creator/18
  Ground10/1 -> Bus Creator/15
  Ground6/1 -> Bus Creator/11
  Constant/1 -> Bus Creator/1
  Constant1/1 -> Bus Creator/2
  Ground1/1 -> Bus Creator/6
  Ground3/1 -> Bus Creator/8
  Ground12/1 -> Bus Creator/17
  Ground14/1 -> Bus Creator/19
  Ground11/1 -> Bus Creator/16
  Ground15/1 -> Bus Creator/20
  Bus Creator/1 -> obj_HeadingSTD/1

== system MIL4L3_SW6_V1_20220211/CarMaker/VehicleControl/SDFADataLog/Subsystem190 ==
  Bus Creator : BusCreator  Inputs=20
  Constant{,1..3} (4 alike) : Constant  Value=0.01
  Ground{,1..15} (16 alike) : Ground
  obj_TTIPCSTD : Outport
  wires:
  Constant2/1 -> Bus Creator/3
  Ground8/1 -> Bus Creator/13
  Ground5/1 -> Bus Creator/10
  Ground9/1 -> Bus Creator/14
  Ground4/1 -> Bus Creator/9
  Constant3/1 -> Bus Creator/4
  Ground7/1 -> Bus Creator/12
  Ground/1 -> Bus Creator/5
  Ground2/1 -> Bus Creator/7
  Ground13/1 -> Bus Creator/18
  Ground10/1 -> Bus Creator/15
  Ground6/1 -> Bus Creator/11
  Constant/1 -> Bus Creator/1
  Constant1/1 -> Bus Creator/2
  Ground1/1 -> Bus Creator/6
  Ground3/1 -> Bus Creator/8
  Ground12/1 -> Bus Creator/17
  Ground14/1 -> Bus Creator/19
  Ground11/1 -> Bus Creator/16
  Ground15/1 -> Bus Creator/20
  Bus Creator/1 -> obj_TTIPCSTD/1

== system MIL4L3_SW6_V1_20220211/CarMaker/VehicleControl/SDFADataLog/Subsystem191 ==
  Bus Creator : BusCreator  Inputs=20
  Constant{,1..3} (4 alike) : Constant  Value=0.01
  Ground{,1..15} (16 alike) : Ground
  obj_PhiBottomSTD : Outport
  wires:
  Bus Creator/1 -> obj_PhiBottomSTD/1
  Ground15/1 -> Bus Creator/20
  Ground11/1 -> Bus Creator/16
  Ground14/1 -> Bus Creator/19
  Ground12/1 -> Bus Creator/17
  Ground3/1 -> Bus Creator/8
  Ground1/1 -> Bus Creator/6
  Constant1/1 -> Bus Creator/2
  Constant/1 -> Bus Creator/1
  Ground6/1 -> Bus Creator/11
  Ground10/1 -> Bus Creator/15
  Ground13/1 -> Bus Creator/18
  Ground2/1 -> Bus Creator/7
  Ground/1 -> Bus Creator/5
  Ground7/1 -> Bus Creator/12
  Constant3/1 -> Bus Creator/4
  Ground4/1 -> Bus Creator/9
  Ground9/1 -> Bus Creator/14
  Ground5/1 -> Bus Creator/10
  Ground8/1 -> Bus Creator/13
  Constant2/1 -> Bus Creator/3

== system MIL4L3_SW6_V1_20220211/CarMaker/VehicleControl/SDFADataLog/Subsystem192 ==
  Bus Creator : BusCreator  Inputs=20
  Ground{,1..15} (16 alike) : Ground
  Read CM Dict : CarMaker4SL/Read CM Dict  xname=User.IO.Out.IFC_obj01_Rel_Vy  xsync=off
  Read CM Dict1 : CarMaker4SL/Read CM Dict  xname=User.IO.Out.IFC_obj02_Rel_Vy  xsync=off
  Read CM Dict2 : CarMaker4SL/Read CM Dict  xname=User.IO.Out.IFC_obj03_Rel_Vy  xsync=off
  Read CM Dict3 : CarMaker4SL/Read CM Dict  xname=User.IO.Out.IFC_obj04_Rel_Vy  xsync=off
  obj_Rel_Vy : Outport
  wires:
  Bus Creator/1 -> obj_Rel_Vy/1
  Ground15/1 -> Bus Creator/20
  Ground11/1 -> Bus Creator/16
  Ground14/1 -> Bus Creator/19
  Ground12/1 -> Bus Creator/17
  Ground3/1 -> Bus Creator/8
  Ground1/1 -> Bus Creator/6
  Read CM Dict1/1 -> Bus Creator/2
  Read CM Dict/1 -> Bus Creator/1
  Ground6/1 -> Bus Creator/11
  Ground10/1 -> Bus Creator/15
  Ground13/1 -> Bus Creator/18
  Ground2/1 -> Bus Creator/7
  Ground/1 -> Bus Creator/5
  Ground7/1 -> Bus Creator/12
  Read CM Dict3/1 -> Bus Creator/4
  Ground4/1 -> Bus Creator/9
  Ground9/1 -> Bus Creator/14
  Ground5/1 -> Bus Creator/10
  Ground8/1 -> Bus Creator/13
  Read CM Dict2/1 -> Bus Creator/3

== system MIL4L3_SW6_V1_20220211/CarMaker/VehicleControl/SDFADataLog/Subsystem193 ==
  Bus Creator : BusCreator  Inputs=20
  Constant{,1..3} (4 alike) : Constant  Value=0.1
  Ground{,1..15} (16 alike) : Ground
  obj_DxSTD : Outport
  wires:
  Constant2/1 -> Bus Creator/3
  Ground8/1 -> Bus Creator/13
  Ground5/1 -> Bus Creator/10
  Ground9/1 -> Bus Creator/14
  Ground4/1 -> Bus Creator/9
  Constant3/1 -> Bus Creator/4
  Ground7/1 -> Bus Creator/12
  Ground/1 -> Bus Creator/5
  Ground2/1 -> Bus Creator/7
  Ground13/1 -> Bus Creator/18
  Ground10/1 -> Bus Creator/15
  Ground6/1 -> Bus Creator/11
  Constant/1 -> Bus Creator/1
  Constant1/1 -> Bus Creator/2
  Ground1/1 -> Bus Creator/6
  Ground3/1 -> Bus Creator/8
  Ground12/1 -> Bus Creator/17
  Ground14/1 -> Bus Creator/19
  Ground11/1 -> Bus Creator/16
  Ground15/1 -> Bus Creator/20
  Bus Creator/1 -> obj_DxSTD/1

== system MIL4L3_SW6_V1_20220211/CarMaker/VehicleControl/SDFADataLog/Subsystem194 ==
  Bus Creator : BusCreator  Inputs=20
  Constant{,1..3} (4 alike) : Constant  Value=0.1
  Ground{,1..15} (16 alike) : Ground
  obj_DySTD : Outport
  wires:
  Constant2/1 -> Bus Creator/3
  Ground8/1 -> Bus Creator/13
  Ground5/1 -> Bus Creator/10
  Ground9/1 -> Bus Creator/14
  Ground4/1 -> Bus Creator/9
  Constant3/1 -> Bus Creator/4
  Ground7/1 -> Bus Creator/12
  Ground/1 -> Bus Creator/5
  Ground2/1 -> Bus Creator/7
  Ground13/1 -> Bus Creator/18
  Ground10/1 -> Bus Creator/15
  Ground6/1 -> Bus Creator/11
  Constant/1 -> Bus Creator/1
  Constant1/1 -> Bus Creator/2
  Ground1/1 -> Bus Creator/6
  Ground3/1 -> Bus Creator/8
  Ground12/1 -> Bus Creator/17
  Ground14/1 -> Bus Creator/19
  Ground11/1 -> Bus Creator/16
  Ground15/1 -> Bus Creator/20
  Bus Creator/1 -> obj_DySTD/1

== system MIL4L3_SW6_V1_20220211/CarMaker/VehicleControl/SDFADataLog/Subsystem195 ==
  Bus Creator : BusCreator  Inputs=20
  Constant{,1..3} (4 alike) : Constant  Value=0.01
  Ground{,1..15} (16 alike) : Ground
  obj_PhiLeftSTD : Outport
  wires:
  Constant2/1 -> Bus Creator/3
  Ground8/1 -> Bus Creator/13
  Ground5/1 -> Bus Creator/10
  Ground9/1 -> Bus Creator/14
  Ground4/1 -> Bus Creator/9
  Constant3/1 -> Bus Creator/4
  Ground7/1 -> Bus Creator/12
  Ground/1 -> Bus Creator/5
  Ground2/1 -> Bus Creator/7
  Ground13/1 -> Bus Creator/18
  Ground10/1 -> Bus Creator/15
  Ground6/1 -> Bus Creator/11
  Constant/1 -> Bus Creator/1
  Constant1/1 -> Bus Creator/2
  Ground1/1 -> Bus Creator/6
  Ground3/1 -> Bus Creator/8
  Ground12/1 -> Bus Creator/17
  Ground14/1 -> Bus Creator/19
  Ground11/1 -> Bus Creator/16
  Ground15/1 -> Bus Creator/20
  Bus Creator/1 -> obj_PhiLeftSTD/1

== system MIL4L3_SW6_V1_20220211/CarMaker/VehicleControl/SDFADataLog/Subsystem196 ==
  Bus Creator : BusCreator  Inputs=20
  Constant{,1..3} (4 alike) : Constant  Value=0.01
  Ground{,1..15} (16 alike) : Ground
  obj_abs_AxSTD : Outport
  wires:
  Constant2/1 -> Bus Creator/3
  Ground8/1 -> Bus Creator/13
  Ground5/1 -> Bus Creator/10
  Ground9/1 -> Bus Creator/14
  Ground4/1 -> Bus Creator/9
  Constant3/1 -> Bus Creator/4
  Ground7/1 -> Bus Creator/12
  Ground/1 -> Bus Creator/5
  Ground2/1 -> Bus Creator/7
  Ground13/1 -> Bus Creator/18
  Ground10/1 -> Bus Creator/15
  Ground6/1 -> Bus Creator/11
  Constant/1 -> Bus Creator/1
  Constant1/1 -> Bus Creator/2
  Ground1/1 -> Bus Creator/6
  Ground3/1 -> Bus Creator/8
  Ground12/1 -> Bus Creator/17
  Ground14/1 -> Bus Creator/19
  Ground11/1 -> Bus Creator/16
  Ground15/1 -> Bus Creator/20
  Bus Creator/1 -> obj_abs_AxSTD/1

== system MIL4L3_SW6_V1_20220211/CarMaker/VehicleControl/SDFADataLog/Subsystem197 ==
  Bus Creator : BusCreator  Inputs=20
  Constant{,1..3} (4 alike) : Constant  Value=0.01
  Ground{,1..15} (16 alike) : Ground
  obj_abs_AySTD : Outport
  wires:
  Constant2/1 -> Bus Creator/3
  Ground8/1 -> Bus Creator/13
  Ground5/1 -> Bus Creator/10
  Ground9/1 -> Bus Creator/14
  Ground4/1 -> Bus Creator/9
  Constant3/1 -> Bus Creator/4
  Ground7/1 -> Bus Creator/12
  Ground/1 -> Bus Creator/5
  Ground2/1 -> Bus Creator/7
  Ground13/1 -> Bus Creator/18
  Ground10/1 -> Bus Creator/15
  Ground6/1 -> Bus Creator/11
  Constant/1 -> Bus Creator/1
  Constant1/1 -> Bus Creator/2
  Ground1/1 -> Bus Creator/6
  Ground3/1 -> Bus Creator/8
  Ground12/1 -> Bus Creator/17
  Ground14/1 -> Bus Creator/19
  Ground11/1 -> Bus Creator/16
  Ground15/1 -> Bus Creator/20
  Bus Creator/1 -> obj_abs_AySTD/1

== system MIL4L3_SW6_V1_20220211/CarMaker/VehicleControl/SDFADataLog/Subsystem198 ==
  Bus Creator : BusCreator  Inputs=20
  Constant{,1..3} (4 alike) : Constant  Value=0.1
  Ground{,1..15} (16 alike) : Ground
  obj_Rel_VxSTD : Outport
  wires:
  Constant2/1 -> Bus Creator/3
  Ground8/1 -> Bus Creator/13
  Ground5/1 -> Bus Creator/10
  Ground9/1 -> Bus Creator/14
  Ground4/1 -> Bus Creator/9
  Constant3/1 -> Bus Creator/4
  Ground7/1 -> Bus Creator/12
  Ground/1 -> Bus Creator/5
  Ground2/1 -> Bus Creator/7
  Ground13/1 -> Bus Creator/18
  Ground10/1 -> Bus Creator/15
  Ground6/1 -> Bus Creator/11
  Constant/1 -> Bus Creator/1
  Constant1/1 -> Bus Creator/2
  Ground1/1 -> Bus Creator/6
  Ground3/1 -> Bus Creator/8
  Ground12/1 -> Bus Creator/17
  Ground14/1 -> Bus Creator/19
  Ground11/1 -> Bus Creator/16
  Ground15/1 -> Bus Creator/20
  Bus Creator/1 -> obj_Rel_VxSTD/1

== system MIL4L3_SW6_V1_20220211/CarMaker/VehicleControl/SDFADataLog/Subsystem199 ==
  Bus Creator : BusCreator  Inputs=20
  Constant{,1..3} (4 alike) : Constant  Value=0.1
  Ground{,1..15} (16 alike) : Ground
  obj_Rel_VySTD : Outport
  wires:
  Constant2/1 -> Bus Creator/3
  Ground8/1 -> Bus Creator/13
  Ground5/1 -> Bus Creator/10
  Ground9/1 -> Bus Creator/14
  Ground4/1 -> Bus Creator/9
  Constant3/1 -> Bus Creator/4
  Ground7/1 -> Bus Creator/12
  Ground/1 -> Bus Creator/5
  Ground2/1 -> Bus Creator/7
  Ground13/1 -> Bus Creator/18
  Ground10/1 -> Bus Creator/15
  Ground6/1 -> Bus Creator/11
  Constant/1 -> Bus Creator/1
  Constant1/1 -> Bus Creator/2
  Ground1/1 -> Bus Creator/6
  Ground3/1 -> Bus Creator/8
  Ground12/1 -> Bus Creator/17
  Ground14/1 -> Bus Creator/19
  Ground11/1 -> Bus Creator/16
  Ground15/1 -> Bus Creator/20
  Bus Creator/1 -> obj_Rel_VySTD/1

== system MIL4L3_SW6_V1_20220211/CarMaker/VehicleControl/SDFADataLog/Subsystem2 ==
  BusCreator : BusCreator  Inputs=24
  Ground{,1..19} (20 alike) : Ground
  Read CM Dict : CarMaker4SL/Read CM Dict  xname=User.IO.Out.ObjectAge_00  xsync=off
  Read CM Dict1 : CarMaker4SL/Read CM Dict  xname=User.IO.Out.ObjectAge_01  xsync=off
  Read CM Dict2 : CarMaker4SL/Read CM Dict  xname=User.IO.Out.ObjectAge_02  xsync=off
  Read CM Dict3 : CarMaker4SL/Read CM Dict  xname=User.IO.Out.ObjectAge_03  xsync=off
  ObjectAge : Outport
  wires:
  Read CM Dict3/1 -> BusCreator/4
  Ground19/1 -> BusCreator/24
  Ground18/1 -> BusCreator/23
  Ground5/1 -> BusCreator/10
  Ground3/1 -> BusCreator/8
  Ground9/1 -> BusCreator/14
  BusCreator/1 -> ObjectAge/1
  Ground11/1 -> BusCreator/16
  Ground8/1 -> BusCreator/13
  Ground7/1 -> BusCreator/12
  Ground15/1 -> BusCreator/18
  Ground1/1 -> BusCreator/6
  Ground/1 -> BusCreator/5
  Ground13/1 -> BusCreator/22
  Ground4/1 -> BusCreator/9
  Ground17/1 -> BusCreator/20
  Read CM Dict/1 -> BusCreator/1
  Ground10/1 -> BusCreator/15
  Read CM Dict2/1 -> BusCreator/3
  Ground6/1 -> BusCreator/11
  Read CM Dict1/1 -> BusCreator/2
  Ground2/1 -> BusCreator/7
  Ground14/1 -> BusCreator/17
  Ground16/1 -> BusCreator/19
  Ground12/1 -> BusCreator/21

== system MIL4L3_SW6_V1_20220211/CarMaker/VehicleControl/SDFADataLog/Subsystem20 ==
  Data Type Conversion7 : DataTypeConversion
  Gain10 : Gain  Gain=180/pi
  Read CM Dict26 : CarMaker4SL/Read CM Dict  xname=Car.YawRate  xsync=off
  Yaw_speed3 : Saturate  UpperLimit=100  LowerLimit=-100
  Yaw_speed : Outport
  wires:
  Gain10/1 -> Yaw_speed3/1  "Yaw_speed"
  Data Type Conversion7/1 -> Yaw_speed/1  "Yaw_speed"
  Yaw_speed3/1 -> Data Type Conversion7/1  "Yaw_speed"
  Read CM Dict26/1 -> Gain10/1  "ESC_YawRate"

== system MIL4L3_SW6_V1_20220211/CarMaker/VehicleControl/SDFADataLog/Subsystem200 ==
  Bus Creator : BusCreator  Inputs=20
  Constant{,1..3} (4 alike) : Constant  Value=0.01
  Ground{,1..15} (16 alike) : Ground
  obj_abgle_3DSTD : Outport
  wires:
  Constant2/1 -> Bus Creator/3
  Ground8/1 -> Bus Creator/13
  Ground5/1 -> Bus Creator/10
  Ground9/1 -> Bus Creator/14
  Ground4/1 -> Bus Creator/9
  Constant3/1 -> Bus Creator/4
  Ground7/1 -> Bus Creator/12
  Ground/1 -> Bus Creator/5
  Ground2/1 -> Bus Creator/7
  Ground13/1 -> Bus Creator/18
  Ground10/1 -> Bus Creator/15
  Ground6/1 -> Bus Creator/11
  Constant/1 -> Bus Creator/1
  Constant1/1 -> Bus Creator/2
  Ground1/1 -> Bus Creator/6
  Ground3/1 -> Bus Creator/8
  Ground12/1 -> Bus Creator/17
  Ground14/1 -> Bus Creator/19
  Ground11/1 -> Bus Creator/16
  Ground15/1 -> Bus Creator/20
  Bus Creator/1 -> obj_abgle_3DSTD/1

== system MIL4L3_SW6_V1_20220211/CarMaker/VehicleControl/SDFADataLog/Subsystem201 ==
  BusCreator : BusCreator  Inputs=24
  Ground{,1..19} (20 alike) : Ground
  Read CM Dict : CarMaker4SL/Read CM Dict  xname=User.IO.Out.AbsoluteLatAcc_00  xsync=off
  Read CM Dict1 : CarMaker4SL/Read CM Dict  xname=User.IO.Out.AbsoluteLatAcc_01  xsync=off
  Read CM Dict2 : CarMaker4SL/Read CM Dict  xname=User.IO.Out.AbsoluteLatAcc_02  xsync=off
  Read CM Dict3 : CarMaker4SL/Read CM Dict  xname=User.IO.Out.AbsoluteLatAcc_03  xsync=off
  AbsoluteLatAcc : Outport
  wires:
  Ground12/1 -> BusCreator/21
  Ground16/1 -> BusCreator/19
  Ground14/1 -> BusCreator/17
  Ground2/1 -> BusCreator/7
  Read CM Dict1/1 -> BusCreator/2
  Ground6/1 -> BusCreator/11
  Read CM Dict2/1 -> BusCreator/3
  Ground10/1 -> BusCreator/15
  Read CM Dict/1 -> BusCreator/1
  Ground17/1 -> BusCreator/20
  Ground4/1 -> BusCreator/9
  Ground13/1 -> BusCreator/22
  Ground/1 -> BusCreator/5
  Ground1/1 -> BusCreator/6
  Ground15/1 -> BusCreator/18
  Ground7/1 -> BusCreator/12
  Ground8/1 -> BusCreator/13
  Ground11/1 -> BusCreator/16
  BusCreator/1 -> AbsoluteLatAcc/1
  Ground9/1 -> BusCreator/14
  Ground3/1 -> BusCreator/8
  Ground5/1 -> BusCreator/10
  Ground18/1 -> BusCreator/23
  Ground19/1 -> BusCreator/24
  Read CM Dict3/1 -> BusCreator/4
